simulink model "lin_modell_test"  (R2016b)
settings: Solver=FixedStepAuto  StartTime=0.0  StopTime=30  FixedStep=0.1  RelTol=1e-3
values from neighbouring files (symbols this model uses):
  st1 = 1    [modell_parameter.m]
undefined symbols (not defined in the file or in its folder): param
settings Model: Creator=Fritz  LastModifiedBy=Fritz

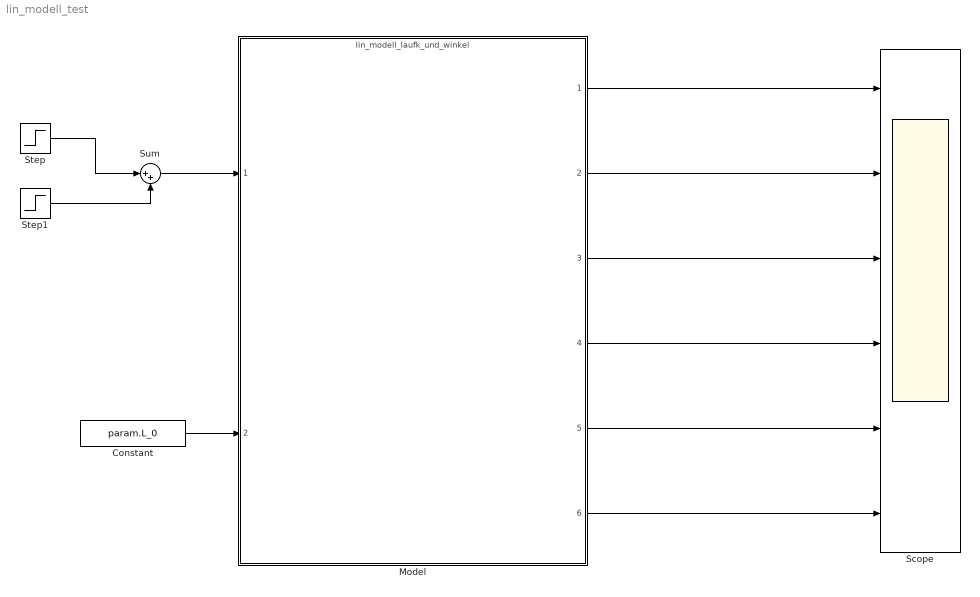
== system lin_modell_test ==
  Constant : Constant  Value=param.L_0
  Model : ModelReference  ModelNameDialog=lin_modell_laufk_und_winkel.slx  SimulationMode=Normal  ModelReferenceVersion=1.38
  Scope : Scope  NumInputPorts=6
  Step : Step  After=st1  SampleTime=0
  Step1 : Step  Time=10  After=-st1  SampleTime=0
  Sum : Sum  Inputs=|++
  wires:
  Model/1 -> Scope/1
  Model/2 -> Scope/2
  Model/3 -> Scope/3
  Model/4 -> Scope/4
  Model/5 -> Scope/5
  Model/6 -> Scope/6
  Step/1 -> Sum/1
  Step1/1 -> Sum/2
  Sum/1 -> Model/1
  Constant/1 -> Model/2
